simulink model "SFCWTD_sim"  (R2016b)
settings: Solver=ode4  StartTime=0.0  StopTime=20  FixedStep=0.001  RelTol=1e-3
values from neighbouring files (symbols this model uses):
  x0 = nova_populacao(1,:)    [gasearch.m]
undefined symbols (not defined in the file or in its folder): B, C, f, g, K, M, tauf, taug, tauu, xdot0
settings Model: Creator=danta  LastModifiedBy=Dantas

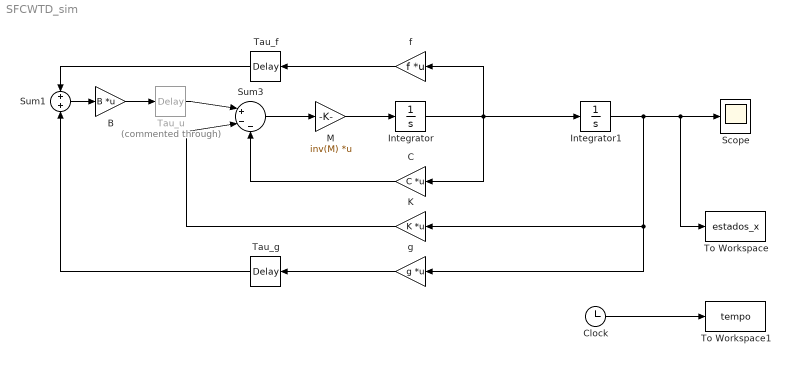
== system SFCWTD_sim ==
  B : Gain  Gain=B  Multiplication=Matrix(K*u)
  C : Gain  Gain=C  Multiplication=Matrix(K*u)
  Clock : Clock
  Integrator : Integrator  InitialCondition=xdot0
  Integrator1 : Integrator  InitialCondition=x0
  K : Gain  Gain=K  Multiplication=Matrix(K*u)
  M : Gain  Gain=inv(M)  Multiplication=Matrix(K*u)
  Scope : Scope
  Sum1 : Sum  Inputs=+|+
  Sum3 : Sum  Inputs=|+--
  Tau_f : TransportDelay  DelayTime=tauf
  Tau_g : TransportDelay  DelayTime=taug
  Tau_u : TransportDelay  Commented=through  DelayTime=tauu
  To Workspace : ToWorkspace  VariableName=estados_x  SampleTime=-1
  To Workspace1 : ToWorkspace  VariableName=tempo  SampleTime=-1
  f : Gain  Gain=f  Multiplication=Matrix(K*u)
  g : Gain  Gain=g  Multiplication=Matrix(K*u)
  wires:
  Sum3/1 -> M/1
  M/1 -> Integrator/1
  Integrator1/1 -> g/1, K/1, To Workspace/1, Scope/1
  Integrator/1 -> f/1, C/1, Integrator1/1
  C/1 -> Sum3/3
  K/1 -> Sum3/2
  Clock/1 -> To Workspace1/1
  g/1 -> Tau_g/1
  Tau_g/1 -> Sum1/2
  f/1 -> Tau_f/1
  Tau_f/1 -> Sum1/1
  Sum1/1 -> B/1
  B/1 -> Tau_u/1
  Tau_u/1 -> Sum3/1
